simulink model "Ode"  (R2020b)
settings: Solver=VariableStepAuto  StartTime=0.0  StopTime=10  RelTol=1e-3
settings Model: Creator=tian  LastModifiedBy=tian

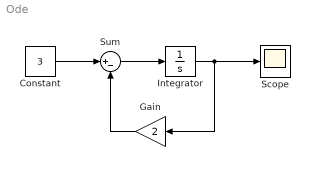
== system Ode ==
  Constant : Constant  Value=3
  Gain : Gain  Gain=2
  Integrator : Integrator  InitialCondition=2
  Scope : Scope
  Sum : Sum  Inputs=|+-
  wires:
  Gain/1 -> Sum/2
  Sum/1 -> Integrator/1
  Integrator/1 -> Gain/1, Scope/1
  Constant/1 -> Sum/1
